simulink model "sistema_completo_lti_simplificado"  (R2019a)
settings: Solver=ode45  StartTime=0.0  StopTime=1.0  MaxStep=1e-6  RelTol=1e-6
undefined symbols (not defined in the file): alpha_cu, b_eq, C_ts, dT_l, J_eq, L_d, L_ls, L_q, lambda_m, P_p, r, R_s_40, R_ts_amb
libraries: eeTransforms x5, simulink x3
settings Model: Creator=pedro  LastModifiedBy=pedro

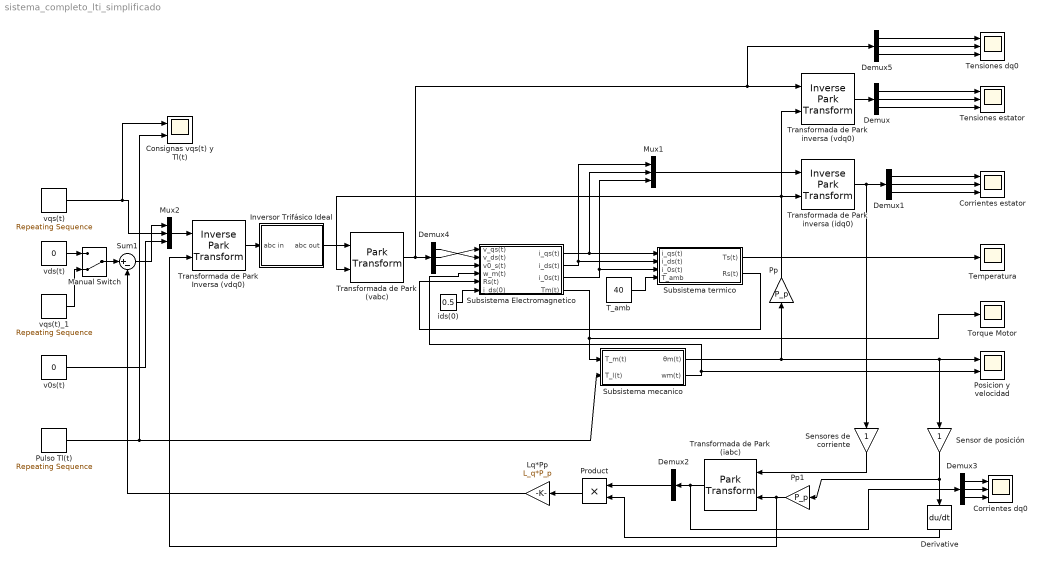
== system sistema_completo_lti_simplificado ==
  Consignas vqs(t) y Tl(t) : Scope  NumInputPorts=2
  Corrientes estator : Scope  NumInputPorts=3
  Corrientes dq0 : Scope  NumInputPorts=3
  Demux{,1..5} (6 alike) : Demux  Outputs=3
  Derivative : Derivative
  Inversor Trifásico Ideal : Subsystem
  Lq*Pp : Gain  Gain=L_q*P_p
  Manual Switch : ManualSwitch  CurrentSetting=0
  Mux1 : Mux  Inputs=3
  Mux2 : Mux  Inputs=3
  Posicion y velocidad : Scope  NumInputPorts=2
  Pp : Gain  Gain=P_p
  Pp1 : Gain  Gain=P_p
  Product : Product
  Pulso Tl(t) : simulink/Sources/Repeating Sequence  rep_seq_t=[0 0.299 0.3 0.499 0.5 0.899 0.9 10]  rep_seq_y=[0 0 dT_l dT_l -dT_l -dT_l 0 0]
  Sensor de posición : Gain
  Sensores de corriente : Gain
  Subsistema Electromagnetico : Subsystem
  "Subsistema mecanico " : Subsystem
  "Subsistema termico " : Subsystem
  Sum1 : Sum  Inputs=|+-
  T_amb : Constant  Value=40
  Temperatura : Scope
  Tensiones estator : Scope  NumInputPorts=3
  Tensiones dq0 : Scope  NumInputPorts=3
  Torque Motor : Scope
  Transformada de Park (iabc) : eeTransforms/Park Transform  AxisAlignment=Q-axis  PowerInvariant=off
      settings: SourceProductName=Simscape Electrical
  "Transformada de Park (vabc) " : eeTransforms/Park Transform  AxisAlignment=Q-axis  PowerInvariant=off
      settings: SourceProductName=Simscape Electrical
  Transformada de Park Inversa (vdq0) : eeTransforms/Inverse Park Transform  AxisAlignment=Q-axis  PowerInvariant=off
      settings: SourceProductName=Simscape Electrical
  Transformada de Park inversa (idq0) : eeTransforms/Inverse Park Transform  AxisAlignment=Q-axis  PowerInvariant=off
      settings: SourceProductName=Simscape Electrical
  "Transformada de Park inversa (vdq0) " : eeTransforms/Inverse Park Transform  AxisAlignment=Q-axis  PowerInvariant=off
      settings: SourceProductName=Simscape Electrical
  ids(0) : Constant  Value=0.5
  v0s(t) : Constant  Value=0
  vds(t) : Constant  Value=0
  vqs(t) : simulink/Sources/Repeating Sequence  rep_seq_t=[0 0.099 0.1 0.699 0.7 10]  rep_seq_y=[0 0 19.596 19.596 0 0]
  vqs(t)_1 : simulink/Sources/Repeating Sequence  rep_seq_t=[0 0.499 0.5 1]  rep_seq_y=[0 0 -1.9596 -1.9596]
  wires:
  Demux5/3 -> Tensiones dq0/3
  Demux5/2 -> Tensiones dq0/2
  ids(0)/1 -> Subsistema Electromagnetico/6(i_ds(0))
  Demux4/2 -> Subsistema Electromagnetico/1(v_qs(t))
  "Subsistema termico "/1(Ts(t)) -> Temperatura/1
  Subsistema Electromagnetico/2(i_ds(t)) -> Mux1/1, "Subsistema termico "/2("i_ds(t) ")
  Demux1/3 -> Corrientes estator/3
  Inversor Trifásico Ideal/1(abc out) -> "Transformada de Park (vabc) "/1
  v0s(t)/1 -> Mux2/3
  Mux2/1 -> Transformada de Park Inversa (vdq0)/1
  Sensor de posición/1 -> Derivative/1, Pp1/1
  Derivative/1 -> Product/2
  Subsistema Electromagnetico/3("i_0s(t) ") -> Mux1/3, "Subsistema termico "/3(i_0s(t))
  Demux1/1 -> Corrientes estator/1
  Demux1/2 -> Corrientes estator/2
  Transformada de Park Inversa (vdq0)/1 -> Inversor Trifásico Ideal/1(abc in)
  Demux2/2 -> Product/1
  Product/1 -> Lq*Pp/1
  Demux/3 -> Tensiones estator/3
  Demux3/1 -> Corrientes dq0/1
  "Transformada de Park inversa (vdq0) "/1 -> Demux/1
  Demux/2 -> Tensiones estator/2
  Demux5/1 -> Tensiones dq0/1
  "Subsistema mecanico "/1(θm(t)) -> Pp/1, Sensor de posición/1, Posicion y velocidad/1
  Pp/1 -> "Transformada de Park (vabc) "/2, Transformada de Park inversa (idq0)/2, "Transformada de Park inversa (vdq0) "/2
  "Subsistema mecanico "/2(wm(t)) -> Posicion y velocidad/2, Subsistema Electromagnetico/4(w_m(t))
  "Subsistema termico "/2(Rs(t)) -> Subsistema Electromagnetico/5("Rs(t) ")
  vqs(t)/1 -> Mux2/2, Consignas vqs(t) y Tl(t)/1
  T_amb/1 -> "Subsistema termico "/4(T_amb)
  Demux4/3 -> Subsistema Electromagnetico/3(v0_s(t))
  Demux3/3 -> Corrientes dq0/3
  Lq*Pp/1 -> Sum1/2
  Sensores de corriente/1 -> Transformada de Park (iabc)/1
  Pp1/1 -> Transformada de Park Inversa (vdq0)/2, Transformada de Park (iabc)/2
  Transformada de Park inversa (idq0)/1 -> Demux1/1, Sensores de corriente/1
  Demux4/1 -> Subsistema Electromagnetico/2(v_ds(t))
  Mux1/1 -> Transformada de Park inversa (idq0)/1
  Subsistema Electromagnetico/4(Tm(t)) -> Torque Motor/1, "Subsistema mecanico "/1("T_m(t) ")
  Sum1/1 -> Mux2/1
  Transformada de Park (iabc)/1 -> Demux3/1, Demux2/1
  Demux3/2 -> Corrientes dq0/2
  "Transformada de Park (vabc) "/1 -> Demux5/1, "Transformada de Park inversa (vdq0) "/1, Demux4/1
  Pulso Tl(t)/1 -> Consignas vqs(t) y Tl(t)/2, "Subsistema mecanico "/2("T_l(t) ")
  Demux/1 -> Tensiones estator/1
  Subsistema Electromagnetico/1("i_qs(t) ") -> Mux1/2, "Subsistema termico "/1("i_qs(t) ")
  Manual Switch/1 -> Sum1/1
  vds(t)/1 -> Manual Switch/1
  vqs(t)_1/1 -> Manual Switch/2

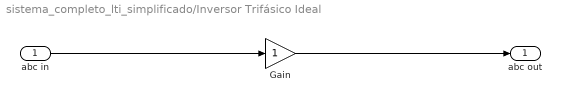
== system sistema_completo_lti_simplificado/Inversor Trifásico Ideal ==
  abc in : Inport
  Gain : Gain
  abc out : Outport
  wires:
  abc in/1 -> Gain/1
  Gain/1 -> abc out/1

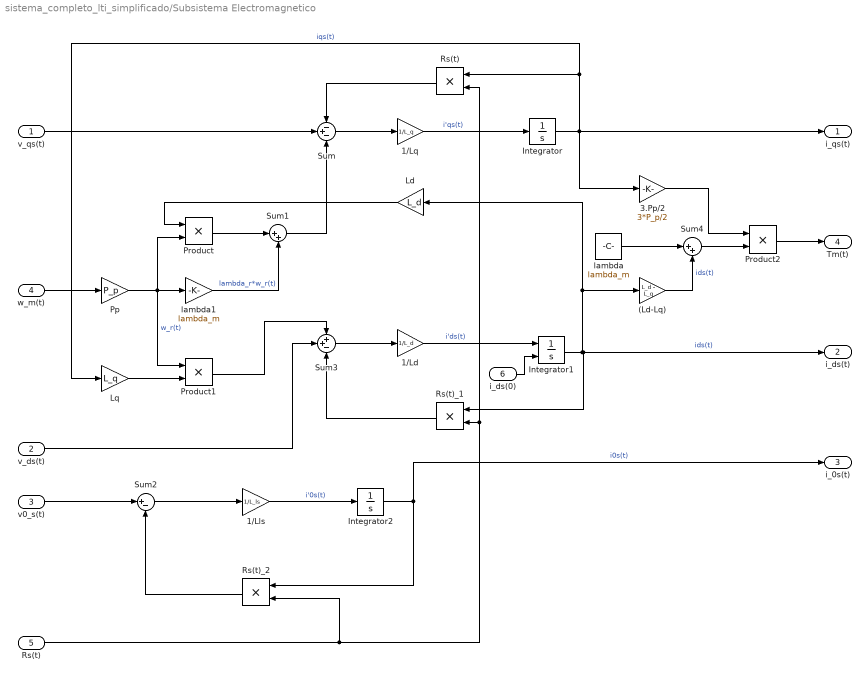
== system sistema_completo_lti_simplificado/Subsistema Electromagnetico ==
  v_qs(t) : Inport
  v_ds(t) : Inport  Port=2
  v0_s(t) : Inport  Port=3
  w_m(t) : Inport  Port=4
  "Rs(t) " : Inport  Port=5
  i_ds(0) : Inport  Port=6
  (Ld-Lq) : Gain  Gain=L_d - L_q
  1/Ld : Gain  Gain=1/L_d
  1/Lls : Gain  Gain=1/L_ls
  1/Lq : Gain  Gain=1/L_q
  3.Pp/2 : Gain  Gain=3*P_p/2
  Integrator : Integrator
  Integrator1 : Integrator  InitialConditionSource=external
  Integrator2 : Integrator
  Ld : Gain  Gain=L_d
  Lq : Gain  Gain=L_q
  Pp : Gain  Gain=P_p
  Product : Product
  Product1 : Product
  Product2 : Product
  Rs(t) : Product
  Rs(t)_1 : Product
  Rs(t)_2 : Product
  Sum : Sum  Inputs=-+-
  Sum1 : Sum  Inputs=|++
  Sum2 : Sum  Inputs=|+-
  Sum3 : Sum  Inputs=++-
  Sum4 : Sum  Inputs=|++
  lambda : Constant  Value=lambda_m
  lambda1 : Gain  Gain=lambda_m
  "i_qs(t) " : Outport
  i_ds(t) : Outport  Port=2
  "i_0s(t) " : Outport  Port=3
  Tm(t) : Outport  Port=4
  wires:
  w_m(t)/1 -> Pp/1
  Pp/1 -> Product1/1, Product/2, lambda1/1  "w_r(t)"
  Sum/1 -> 1/Lq/1
  1/Lq/1 -> Integrator/1  "i'qs(t)"
  Sum1/1 -> Sum/3
  v_qs(t)/1 -> Sum/2
  Integrator/1 -> Lq/1, Rs(t)/1, 3.Pp/2/1, "i_qs(t) "/1  "iqs(t)"
  lambda1/1 -> Sum1/2  "lambda_r*w_r(t)"
  Product/1 -> Sum1/1
  v_ds(t)/1 -> Sum3/2
  Sum3/1 -> 1/Ld/1
  Product1/1 -> Sum3/1
  1/Ld/1 -> Integrator1/1  "i'ds(t)"
  Integrator1/1 -> Ld/1, (Ld-Lq)/1, Rs(t)_1/1, i_ds(t)/1  "ids(t)"
  Lq/1 -> Product1/2
  Ld/1 -> Product/1
  v0_s(t)/1 -> Sum2/1
  Rs(t)_2/1 -> Sum2/2
  Sum2/1 -> 1/Lls/1
  1/Lls/1 -> Integrator2/1  "i'0s(t)"
  Integrator2/1 -> Rs(t)_2/1, "i_0s(t) "/1  "i0s(t)"
  (Ld-Lq)/1 -> Sum4/2  "ids(t)"
  lambda/1 -> Sum4/1
  Sum4/1 -> Product2/2
  Product2/1 -> Tm(t)/1
  3.Pp/2/1 -> Product2/1
  "Rs(t) "/1 -> Rs(t)_2/2, Rs(t)/2, Rs(t)_1/2
  Rs(t)_1/1 -> Sum3/3
  Rs(t)/1 -> Sum/1
  i_ds(0)/1 -> Integrator1/2

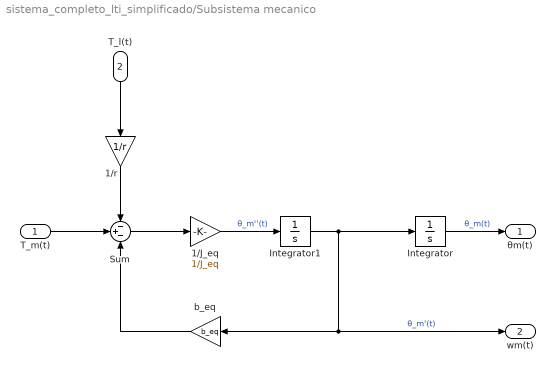
== system sistema_completo_lti_simplificado/Subsistema mecanico  ==
  "T_m(t) " : Inport
  "T_l(t) " : Inport  Port=2
  "1/J_eq " : Gain  Gain=1/J_eq
  1/r : Gain  Gain=1/r
  Integrator : Integrator
  Integrator1 : Integrator
  Sum : Sum  Inputs=-+-
  b_eq : Gain  Gain=b_eq
  θm(t) : Outport
  wm(t) : Outport  Port=2
  wires:
  Integrator1/1 -> b_eq/1, wm(t)/1, Integrator/1  "θ_m'(t)"
  Sum/1 -> "1/J_eq "/1
  b_eq/1 -> Sum/3
  "1/J_eq "/1 -> Integrator1/1  "θ_m''(t)"
  Integrator/1 -> θm(t)/1  "θ_m(t)"
  "T_m(t) "/1 -> Sum/2
  "T_l(t) "/1 -> 1/r/1
  1/r/1 -> Sum/1

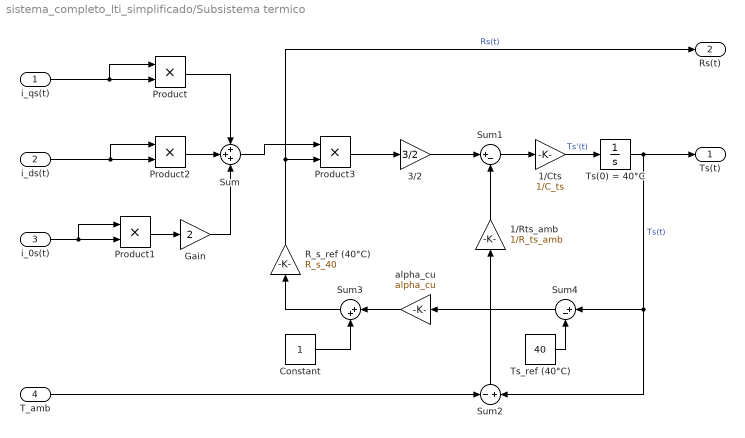
== system sistema_completo_lti_simplificado/Subsistema termico  ==
  "i_qs(t) " : Inport
  "i_ds(t) " : Inport  Port=2
  i_0s(t) : Inport  Port=3
  T_amb : Inport  Port=4
  1/Cts : Gain  Gain=1/C_ts
  1/Rts_amb : Gain  Gain=1/R_ts_amb
  3/2 : Gain  Gain=3/2
  Constant : Constant
  Gain : Gain  Gain=2
  Product{,1..3} (4 alike) : Product
  R_s_ref (40°C) : Gain  Gain=R_s_40
  Sum : Sum  Inputs=+++
  Sum1 : Sum  Inputs=|+-
  Sum2 : Sum  Inputs=-|+
  Sum3 : Sum  Inputs=|++
  Sum4 : Sum  Inputs=|+-
  Ts(0) = 40°C : Integrator  InitialCondition=40
  Ts_ref (40°C) : Constant  Value=40
  alpha_cu : Gain  Gain=alpha_cu
  Ts(t) : Outport
  Rs(t) : Outport  Port=2
  wires:
  i_0s(t)/1 -> Product1/1, Product1/2
  "i_ds(t) "/1 -> Product2/1, Product2/2
  "i_qs(t) "/1 -> Product/1, Product/2
  Product/1 -> Sum/1
  Product2/1 -> Sum/2
  Ts(0) = 40°C/1 -> Sum4/1, Sum2/2, Ts(t)/1  "Ts(t)"
  T_amb/1 -> Sum2/1
  Sum2/1 -> 1/Rts_amb/1
  1/Rts_amb/1 -> Sum1/2
  Sum1/1 -> 1/Cts/1
  1/Cts/1 -> Ts(0) = 40°C/1  "Ts'(t)"
  Constant/1 -> Sum3/2
  alpha_cu/1 -> Sum3/1
  Sum3/1 -> R_s_ref (40°C)/1
  R_s_ref (40°C)/1 -> Rs(t)/1, Product3/2  "Rs(t)"
  Sum/1 -> Product3/1
  Product3/1 -> 3/2/1
  3/2/1 -> Sum1/1
  Ts_ref (40°C)/1 -> Sum4/2
  Sum4/1 -> alpha_cu/1
  Gain/1 -> Sum/3
  Product1/1 -> Gain/1
